simulink library "DSCA"  (R2016b)
settings: Solver=VariableStepAuto  StartTime=0.0  StopTime=10.0  RelTol=1e-3
undefined symbols (not defined in the file): CAL_FilterResetThd, CAL_MeasNoiseVelKF, CAL_mm_PER_tick, CAL_NORTH, CAL_procNoiseVelKF, CAL_ROBO_LENG, CAL_WheelDiameter_cm, CONST_EnableDelay, CONST_EndOfLineEnableFlg, ENU_BACKWARD, ENU_DIAG, ENU_FORWARD, ENU_STOP, gearRatio
libraries: movingAverage_1ms_to_5ms x5, simulink_need_slupdate x2, MotorModelDiscreteTf x2, ThetaOverFlowFilter x1
settings Model: Creator=oelkawok  LastModifiedBy=oelkawok

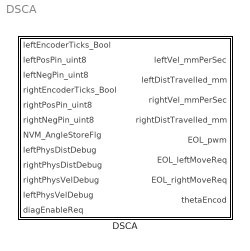
== system DSCA ==
  DSCA : Subsystem  TreatAsAtomicUnit=on

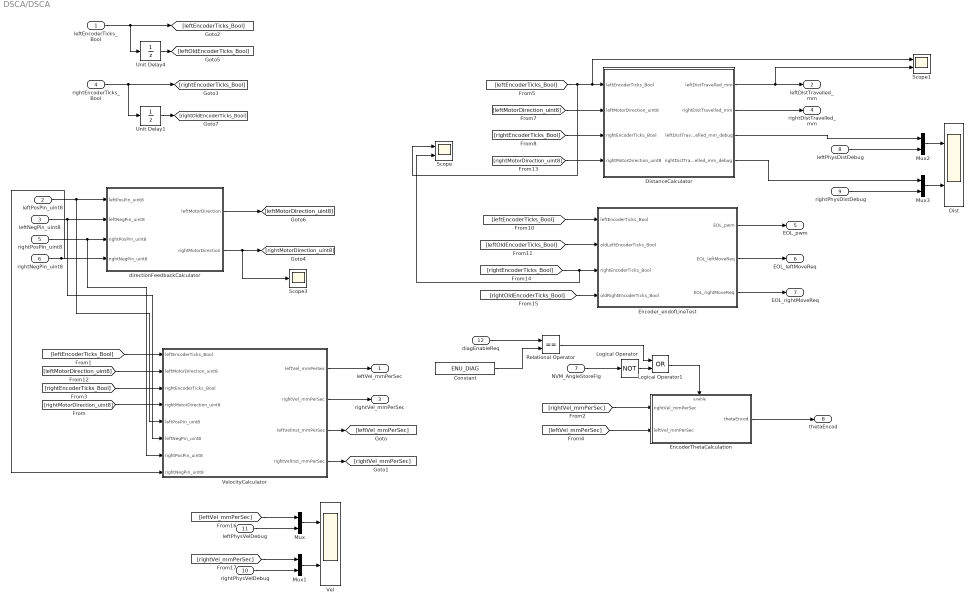
== system DSCA/DSCA ==
  leftEncoderTicks_Bool : Inport
  leftPosPin_uint8 : Inport  Port=2
  leftNegPin_uint8 : Inport  Port=3
  rightEncoderTicks_Bool : Inport  Port=4
  rightPosPin_uint8 : Inport  Port=5
  rightNegPin_uint8 : Inport  Port=6
  NVM_AngleStoreFlg : Inport  Port=7
  leftPhysDistDebug : Inport  Port=8
  rightPhysDistDebug : Inport  Port=9
  rightPhysVelDebug : Inport  Port=10
  leftPhysVelDebug : Inport  Port=11
  diagEnableReq : Inport  Port=12
  Constant : Constant  Value=ENU_DIAG
  Dist : Scope  NumInputPorts=2
  DistanceCalculator : Subsystem
  EncoderThetaCalculation : Subsystem
  Encoder_endofLineTest : Subsystem
  Logical Operator : Logic  Operator=NOT  IconShape=distinctive  AllPortsSameDT=off  OutDataTypeStr=boolean
  Logical Operator1 : Logic  Operator=OR  AllPortsSameDT=off  OutDataTypeStr=boolean
  Mux{,1..3} (4 alike) : Mux  Inputs=2
  Relational Operator : RelationalOperator  Operator===  OutDataTypeStr=boolean  RndMeth=Simplest
  Scope : Scope  NumInputPorts=2
  Scope1 : Scope  NumInputPorts=2
  Scope3 : Scope
  Unit Delay1 : UnitDelay  SampleTime=-1
      settings: AttributesFormatString=Init: %<InitialCondition>
  Unit Delay4 : UnitDelay  SampleTime=-1
      settings: AttributesFormatString=Init: %<InitialCondition>
  Vel : Scope  NumInputPorts=2
  VelocityCalculator : Subsystem
  directionFeedbackCalculator : Subsystem
  leftVel_mmPerSec : Outport
  leftDistTravelled_mm : Outport  Port=2
  rightVel_mmPerSec : Outport  Port=3
  rightDistTravelled_mm : Outport  Port=4
  EOL_pwm : Outport  Port=5
  EOL_leftMoveReq : Outport  Port=6
  EOL_rightMoveReq : Outport  Port=7
  thetaEncod : Outport  Port=8
  wires:
  Relational Operator/1 -> Logical Operator1/1
  Constant/1 -> Relational Operator/2
  diagEnableReq/1 -> Relational Operator/1
  Logical Operator1/1 -> EncoderThetaCalculation/Enable
  Logical Operator/1 -> Logical Operator1/2
  VelocityCalculator/2(rightVel_mmPerSec) -> rightVel_mmPerSec/1
  VelocityCalculator/1(leftVel_mmPerSec) -> leftVel_mmPerSec/1
  EncoderThetaCalculation/1(thetaEncod) -> thetaEncod/1
  rightPhysVelDebug/1 -> Mux1/2
  leftPhysVelDebug/1 -> Mux/2
  [rightVel_mmPerSec] -> Mux1/1
  [leftVel_mmPerSec] -> Mux/1
  [rightVel_mmPerSec] -> EncoderThetaCalculation/1(rightVel_mmPerSec)
  [leftVel_mmPerSec] -> EncoderThetaCalculation/2(leftVel_mmPerSec)
  VelocityCalculator/3(leftVelInst_mmPerSec) -> [leftVel_mmPerSec]
  VelocityCalculator/4(rightVelInst_mmPerSec) -> [rightVel_mmPerSec]
  rightPhysDistDebug/1 -> Mux3/2
  DistanceCalculator/4(rightDistTravelled_mm_debug) -> Mux3/1
  Mux3/1 -> Dist/2
  Mux2/1 -> Dist/1
  [rightMotorDirection_uint8] -> VelocityCalculator/4(rightMotorDirection_uint8)
  Mux1/1 -> Vel/2
  Mux/1 -> Vel/1
  leftPhysDistDebug/1 -> Mux2/2
  DistanceCalculator/3(leftDistTravelled_mm_debug) -> Mux2/1
  NVM_AngleStoreFlg/1 -> Logical Operator/1
  Encoder_endofLineTest/1(EOL_pwm) -> EOL_pwm/1
  Encoder_endofLineTest/2(EOL_leftMoveReq) -> EOL_leftMoveReq/1
  Encoder_endofLineTest/3(EOL_rightMoveReq) -> EOL_rightMoveReq/1
  [rightOldEncoderTicks_Bool] -> Encoder_endofLineTest/4(oldRightEncoderTicks_Bool)
  [rightEncoderTicks_Bool] -> Encoder_endofLineTest/3(rightEncoderTicks_Bool), Scope/2
  [leftOldEncoderTicks_Bool] -> Encoder_endofLineTest/2(oldLeftEncoderTicks_Bool)
  [leftEncoderTicks_Bool] -> Encoder_endofLineTest/1(leftEncoderTicks_Bool)
  [rightEncoderTicks_Bool] -> DistanceCalculator/3(rightEncoderTicks_Bool)
  [leftEncoderTicks_Bool] -> DistanceCalculator/1(leftEncoderTicks_Bool), Scope1/1, Scope/1
  [rightEncoderTicks_Bool] -> VelocityCalculator/3(rightEncoderTicks_Bool)
  [leftEncoderTicks_Bool] -> VelocityCalculator/1(leftEncoderTicks_Bool)
  Unit Delay4/1 -> [leftOldEncoderTicks_Bool]
  Unit Delay1/1 -> [rightOldEncoderTicks_Bool]
  leftEncoderTicks_Bool/1 -> Unit Delay4/1, [leftEncoderTicks_Bool]
  rightEncoderTicks_Bool/1 -> [rightEncoderTicks_Bool], Unit Delay1/1
  [leftMotorDirection_uint8] -> VelocityCalculator/2(leftMotorDirection_uint8)
  DistanceCalculator/2(rightDistTravelled_mm) -> rightDistTravelled_mm/1
  [rightMotorDirection_uint8] -> DistanceCalculator/4(rightMotorDirection_uint8)
  [leftMotorDirection_uint8] -> DistanceCalculator/2(leftMotorDirection_uint8)
  DistanceCalculator/1(leftDistTravelled_mm) -> leftDistTravelled_mm/1, Scope1/2
  directionFeedbackCalculator/2(rightMotorDirection) -> [rightMotorDirection_uint8], Scope3/1
  rightNegPin_uint8/1 -> directionFeedbackCalculator/4(rightNegPin_uint8), VelocityCalculator/8(rightNegPin_uint8)
  rightPosPin_uint8/1 -> directionFeedbackCalculator/3(rightPosPin_uint8), VelocityCalculator/7(rightPosPin_uint8)
  directionFeedbackCalculator/1(leftMotorDirection) -> [leftMotorDirection_uint8]
  leftNegPin_uint8/1 -> directionFeedbackCalculator/2(leftNegPin_uint8), VelocityCalculator/6(leftNegPin_uint8)
  leftPosPin_uint8/1 -> directionFeedbackCalculator/1(leftPosPin_uint8), VelocityCalculator/5(leftPosPin_uint8)

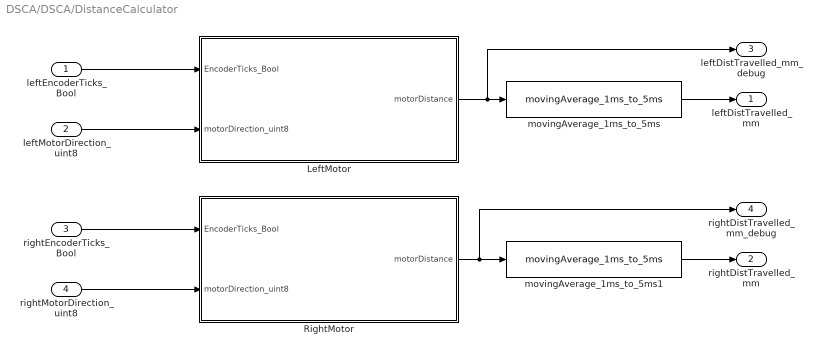
== system DSCA/DSCA/DistanceCalculator ==
  leftEncoderTicks_Bool : Inport
  leftMotorDirection_uint8 : Inport  Port=2
  rightEncoderTicks_Bool : Inport  Port=3
  rightMotorDirection_uint8 : Inport  Port=4
  LeftMotor : Subsystem
  RightMotor : Subsystem
  movingAverage_1ms_to_5ms : movingAverage_1ms_to_5ms/movingAverage_1ms_to_5ms
  movingAverage_1ms_to_5ms1 : movingAverage_1ms_to_5ms/movingAverage_1ms_to_5ms
  leftDistTravelled_mm : Outport
  rightDistTravelled_mm : Outport  Port=2
  leftDistTravelled_mm_debug : Outport  Port=3
  rightDistTravelled_mm_debug : Outport  Port=4
  wires:
  rightMotorDirection_uint8/1 -> RightMotor/2(motorDirection_uint8)
  rightEncoderTicks_Bool/1 -> RightMotor/1(EncoderTicks_Bool)
  leftMotorDirection_uint8/1 -> LeftMotor/2(motorDirection_uint8)
  leftEncoderTicks_Bool/1 -> LeftMotor/1(EncoderTicks_Bool)
  movingAverage_1ms_to_5ms/1 -> leftDistTravelled_mm/1
  LeftMotor/1(motorDistance) -> leftDistTravelled_mm_debug/1, movingAverage_1ms_to_5ms/1
  movingAverage_1ms_to_5ms1/1 -> rightDistTravelled_mm/1
  RightMotor/1(motorDistance) -> rightDistTravelled_mm_debug/1, movingAverage_1ms_to_5ms1/1

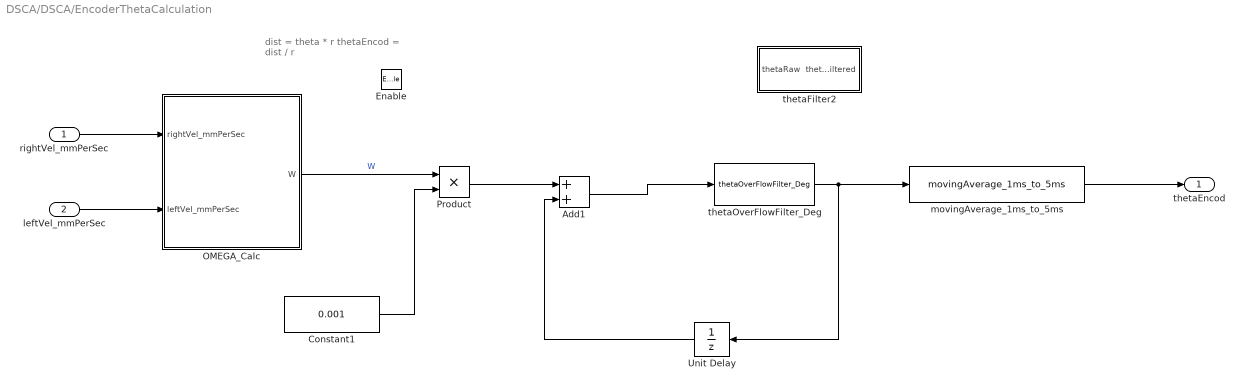
== system DSCA/DSCA/EncoderThetaCalculation ==
  note: dist = theta * r
      | thetaEncod = dist / r
  rightVel_mmPerSec : Inport
  leftVel_mmPerSec : Inport  Port=2
  Enable : EnablePort
  Add1 : Sum
  Constant1 : Constant  Value=0.001
  OMEGA_Calc : Subsystem
  Product : Product
  Unit Delay : UnitDelay  InitialCondition=CAL_NORTH  SampleTime=-1
  movingAverage_1ms_to_5ms : movingAverage_1ms_to_5ms/movingAverage_1ms_to_5ms
  thetaFilter2 : Subsystem
  thetaOverFlowFilter_Deg : ThetaOverFlowFilter/thetaOverFlowFilter_Deg
  thetaEncod : Outport
  wires:
  movingAverage_1ms_to_5ms/1 -> thetaEncod/1
  Unit Delay/1 -> Add1/2
  Add1/1 -> thetaOverFlowFilter_Deg/1
  Product/1 -> Add1/1
  thetaOverFlowFilter_Deg/1 -> Unit Delay/1, movingAverage_1ms_to_5ms/1
  rightVel_mmPerSec/1 -> OMEGA_Calc/1(rightVel_mmPerSec)
  leftVel_mmPerSec/1 -> OMEGA_Calc/2(leftVel_mmPerSec)
  OMEGA_Calc/1(W) -> Product/1  "W"
  Constant1/1 -> Product/2

== system DSCA/DSCA/Encoder_endofLineTest ==
  leftEncoderTicks_Bool : Inport
  oldLeftEncoderTicks_Bool : Inport  Port=2
  rightEncoderTicks_Bool : Inport  Port=3
  oldRightEncoderTicks_Bool : Inport  Port=4
  CONST_EndOfLineEnableFlg : Constant  Value=CONST_EndOfLineEnableFlg
  endofLineTest : Subsystem
  EOL_pwm : Outport
  EOL_leftMoveReq : Outport  Port=2
  EOL_rightMoveReq : Outport  Port=3
  wires:
  endofLineTest/2(EOL_leftMoveReq) -> EOL_leftMoveReq/1
  endofLineTest/3(EOL_rightMoveReq) -> EOL_rightMoveReq/1
  oldRightEncoderTicks_Bool/1 -> endofLineTest/4(oldRightEncoderTicks_Bool)
  rightEncoderTicks_Bool/1 -> endofLineTest/3(rightEncoderTicks_Bool)
  leftEncoderTicks_Bool/1 -> endofLineTest/1(leftEncoderTicks_Bool)
  oldLeftEncoderTicks_Bool/1 -> endofLineTest/2(oldLeftEncoderTicks_Bool)
  endofLineTest/1(EOL_pwm) -> EOL_pwm/1
  CONST_EndOfLineEnableFlg/1 -> endofLineTest/Enable

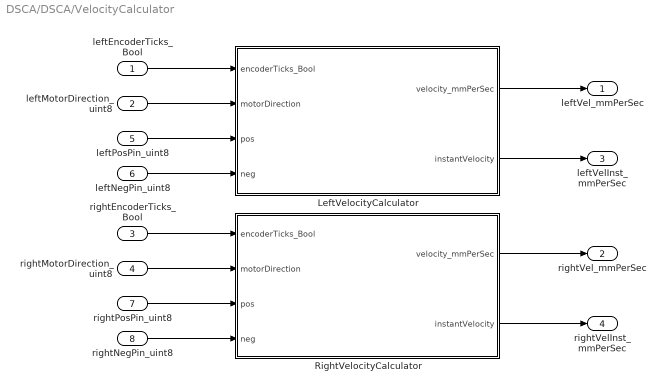
== system DSCA/DSCA/VelocityCalculator ==
  leftEncoderTicks_Bool : Inport
  leftMotorDirection_uint8 : Inport  Port=2
  rightEncoderTicks_Bool : Inport  Port=3
  rightMotorDirection_uint8 : Inport  Port=4
  leftPosPin_uint8 : Inport  Port=5
  leftNegPin_uint8 : Inport  Port=6
  rightPosPin_uint8 : Inport  Port=7
  rightNegPin_uint8 : Inport  Port=8
  LeftVelocityCalculator : Subsystem
  RightVelocityCalculator : Subsystem
  leftVel_mmPerSec : Outport
  rightVel_mmPerSec : Outport  Port=2
  leftVelInst_mmPerSec : Outport  Port=3
  rightVelInst_mmPerSec : Outport  Port=4
  wires:
  rightNegPin_uint8/1 -> RightVelocityCalculator/4(neg)
  rightPosPin_uint8/1 -> RightVelocityCalculator/3(pos)
  leftNegPin_uint8/1 -> LeftVelocityCalculator/4(neg)
  leftPosPin_uint8/1 -> LeftVelocityCalculator/3(pos)
  RightVelocityCalculator/2(instantVelocity) -> rightVelInst_mmPerSec/1
  LeftVelocityCalculator/2(instantVelocity) -> leftVelInst_mmPerSec/1
  leftMotorDirection_uint8/1 -> LeftVelocityCalculator/2(motorDirection)
  rightMotorDirection_uint8/1 -> RightVelocityCalculator/2(motorDirection)
  LeftVelocityCalculator/1(velocity_mmPerSec) -> leftVel_mmPerSec/1
  leftEncoderTicks_Bool/1 -> LeftVelocityCalculator/1(encoderTicks_Bool)
  RightVelocityCalculator/1(velocity_mmPerSec) -> rightVel_mmPerSec/1
  rightEncoderTicks_Bool/1 -> RightVelocityCalculator/1(encoderTicks_Bool)

== system DSCA/DSCA/directionFeedbackCalculator ==
  leftPosPin_uint8 : Inport
  leftNegPin_uint8 : Inport  Port=2
  rightPosPin_uint8 : Inport  Port=3
  rightNegPin_uint8 : Inport  Port=4
  LeftMotor : Subsystem
  RightMotor : Subsystem
  leftMotorDirection : Outport
  rightMotorDirection : Outport  Port=2
  wires:
  RightMotor/1(MotorDirection) -> rightMotorDirection/1
  rightNegPin_uint8/1 -> RightMotor/2(NegPin_uint8)
  rightPosPin_uint8/1 -> RightMotor/1(PosPin_uint8)
  LeftMotor/1(MotorDirection) -> leftMotorDirection/1
  leftNegPin_uint8/1 -> LeftMotor/2(NegPin_uint8)
  leftPosPin_uint8/1 -> LeftMotor/1(PosPin_uint8)

== system DSCA/DSCA/DistanceCalculator/LeftMotor ==
  EncoderTicks_Bool : Inport
  motorDirection_uint8 : Inport  Port=2
  Data Type Conversion : DataTypeConversion  OutDataTypeStr=single
  EncoderIncrement : Subsystem  TreatAsAtomicUnit=on
  Gain1 : Gain  Gain=CAL_mm_PER_tick
  motorDistance : Outport
  wires:
  motorDirection_uint8/1 -> EncoderIncrement/1(motorDirection)
  EncoderTicks_Bool/1 -> EncoderIncrement/Trigger
  EncoderIncrement/1(distCounter) -> Data Type Conversion/1
  Gain1/1 -> motorDistance/1
  Data Type Conversion/1 -> Gain1/1

== system DSCA/DSCA/DistanceCalculator/RightMotor ==
  EncoderTicks_Bool : Inport
  motorDirection_uint8 : Inport  Port=2
  Data Type Conversion : DataTypeConversion  OutDataTypeStr=single
  EncoderIncrement : Subsystem  TreatAsAtomicUnit=on
  Gain1 : Gain  Gain=CAL_mm_PER_tick
  motorDistance : Outport
  wires:
  Data Type Conversion/1 -> Gain1/1
  Gain1/1 -> motorDistance/1
  EncoderIncrement/1(distCounter) -> Data Type Conversion/1
  EncoderTicks_Bool/1 -> EncoderIncrement/Trigger
  motorDirection_uint8/1 -> EncoderIncrement/1(motorDirection)

== system DSCA/DSCA/EncoderThetaCalculation/OMEGA_Calc ==
  rightVel_mmPerSec : Inport
  leftVel_mmPerSec : Inport  Port=2
  Add : Sum  Inputs=+-
  Constant3 : Constant  Value=CAL_ROBO_LENG
  Divide1 : Product  Inputs=*/  OutDataTypeStr=single
  W : Outport
  wires:
  rightVel_mmPerSec/1 -> Add/2
  leftVel_mmPerSec/1 -> Add/1
  Add/1 -> Divide1/1
  Divide1/1 -> W/1
  Constant3/1 -> Divide1/2

== system DSCA/DSCA/EncoderThetaCalculation/thetaFilter2 ==
  thetaRaw : Inport
  Add : Sum  Inputs=+-
  Add1 : Sum
  Constant : Constant  Value=360
  Constant1 : Constant  Value=360
  Constant2 : Constant  Value=0
  Relational Operator : RelationalOperator  Operator=>  OutDataTypeStr=boolean  RndMeth=Nearest
  Relational Operator1 : RelationalOperator  Operator=<  OutDataTypeStr=boolean  RndMeth=Nearest
  Switch : Switch  Criteria=u2 > Threshold
  Switch1 : Switch  Criteria=u2 > Threshold
  thetaFiltered : Outport
  wires:
  thetaRaw/1 -> Switch1/3, Add/1, Add1/2, Relational Operator1/1, Relational Operator/1
  Constant/1 -> Add1/1, Relational Operator/2
  Relational Operator/1 -> Switch/2
  Constant1/1 -> Add/2
  Add/1 -> Switch/1
  Constant2/1 -> Relational Operator1/2
  Relational Operator1/1 -> Switch1/2
  Add1/1 -> Switch1/1
  Switch1/1 -> Switch/3
  Switch/1 -> thetaFiltered/1

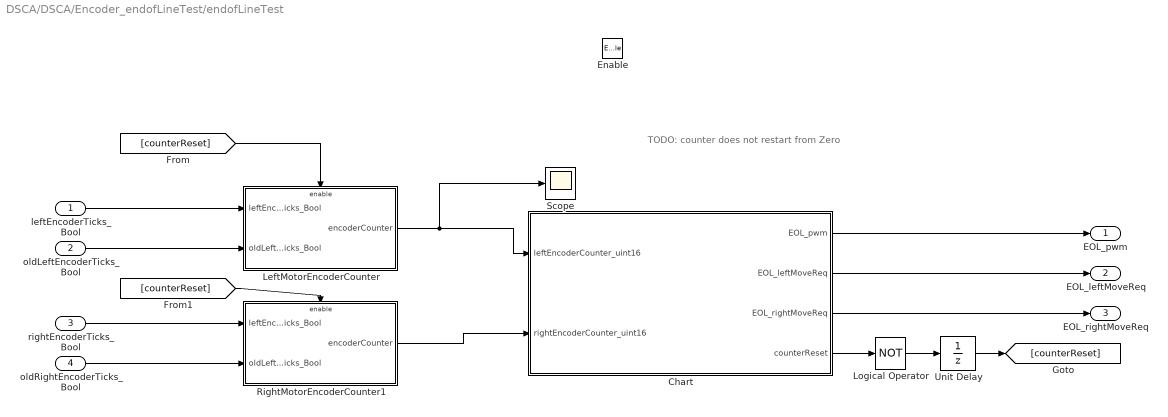
== system DSCA/DSCA/Encoder_endofLineTest/endofLineTest ==
  note: TODO: counter does not restart from Zero
  leftEncoderTicks_Bool : Inport
  oldLeftEncoderTicks_Bool : Inport  Port=2
  rightEncoderTicks_Bool : Inport  Port=3
  oldRightEncoderTicks_Bool : Inport  Port=4
  Enable : EnablePort
  Chart : Stateflow chart  TreatAsAtomicUnit=on
  LeftMotorEncoderCounter : Subsystem
  Logical Operator : Logic  Operator=NOT  Inputs=NOT  IconShape=distinctive  AllPortsSameDT=off  OutDataTypeStr=boolean
  RightMotorEncoderCounter1 : Subsystem
  Scope : Scope
  Unit Delay : UnitDelay  InitialCondition=1  SampleTime=-1
  EOL_pwm : Outport
  EOL_leftMoveReq : Outport  Port=2
  EOL_rightMoveReq : Outport  Port=3
  wires:
  LeftMotorEncoderCounter/1(encoderCounter) -> Chart/1(leftEncoderCounter_uint16), Scope/1
  Unit Delay/1 -> [counterReset]
  Chart/3(EOL_rightMoveReq) -> EOL_rightMoveReq/1
  Chart/2(EOL_leftMoveReq) -> EOL_leftMoveReq/1
  Chart/1(EOL_pwm) -> EOL_pwm/1
  Logical Operator/1 -> Unit Delay/1
  [counterReset] -> LeftMotorEncoderCounter/Enable
  [counterReset] -> RightMotorEncoderCounter1/Enable
  Chart/4(counterReset) -> Logical Operator/1
  RightMotorEncoderCounter1/1(encoderCounter) -> Chart/2(rightEncoderCounter_uint16)
  rightEncoderTicks_Bool/1 -> RightMotorEncoderCounter1/1(leftEncoderTicks_Bool)
  oldRightEncoderTicks_Bool/1 -> RightMotorEncoderCounter1/2(oldLeftEncoderTicks_Bool)
  oldLeftEncoderTicks_Bool/1 -> LeftMotorEncoderCounter/2(oldLeftEncoderTicks_Bool)
  leftEncoderTicks_Bool/1 -> LeftMotorEncoderCounter/1(leftEncoderTicks_Bool)

== system DSCA/DSCA/VelocityCalculator/LeftVelocityCalculator ==
  encoderTicks_Bool : Inport
  motorDirection : Inport  Port=2
  pos : Inport  Port=3
  neg : Inport  Port=4
  LeftMotor : Subsystem
  movingAverage_1ms_to_5ms : movingAverage_1ms_to_5ms/movingAverage_1ms_to_5ms
  velocity_mmPerSec : Outport
  instantVelocity : Outport  Port=2
  wires:
  neg/1 -> LeftMotor/4(neg)
  pos/1 -> LeftMotor/3(pos)
  movingAverage_1ms_to_5ms/1 -> velocity_mmPerSec/1
  LeftMotor/1(motorSpd) -> instantVelocity/1, movingAverage_1ms_to_5ms/1
  motorDirection/1 -> LeftMotor/2(motorDirection_uint8)
  encoderTicks_Bool/1 -> LeftMotor/1(EncoderTicks_Bool)

== system DSCA/DSCA/VelocityCalculator/RightVelocityCalculator ==
  encoderTicks_Bool : Inport
  motorDirection : Inport  Port=2
  pos : Inport  Port=3
  neg : Inport  Port=4
  LeftMotor : Subsystem
  movingAverage_1ms_to_5ms : movingAverage_1ms_to_5ms/movingAverage_1ms_to_5ms
  velocity_mmPerSec : Outport
  instantVelocity : Outport  Port=2
  wires:
  neg/1 -> LeftMotor/4(neg)
  pos/1 -> LeftMotor/3(pos)
  movingAverage_1ms_to_5ms/1 -> velocity_mmPerSec/1
  encoderTicks_Bool/1 -> LeftMotor/1(EncoderTicks_Bool)
  LeftMotor/1(motorSpd) -> instantVelocity/1, movingAverage_1ms_to_5ms/1
  motorDirection/1 -> LeftMotor/2(motorDirection_uint8)

== system DSCA/DSCA/directionFeedbackCalculator/LeftMotor ==
  PosPin_uint8 : Inport
  NegPin_uint8 : Inport  Port=2
  Constant13 : Constant  Value=ENU_STOP
  Constant14 : Constant  Value=ENU_BACKWARD
  Constant15 : Constant  Value=ENU_FORWARD
  Relational Operator5 : RelationalOperator  Operator=>  OutDataTypeStr=boolean  RndMeth=Simplest
  Relational Operator6 : RelationalOperator  Operator=<  OutDataTypeStr=boolean  RndMeth=Simplest
  Switch5 : Switch  Criteria=u2 ~= 0
  Switch6 : Switch  Criteria=u2 ~= 0
  MotorDirection : Outport
  wires:
  NegPin_uint8/1 -> Relational Operator5/2, Relational Operator6/2
  Relational Operator5/1 -> Switch5/2
  PosPin_uint8/1 -> Relational Operator5/1, Relational Operator6/1
  Constant14/1 -> Switch6/1
  Constant13/1 -> Switch6/3
  Constant15/1 -> Switch5/1
  Relational Operator6/1 -> Switch6/2
  Switch6/1 -> Switch5/3
  Switch5/1 -> MotorDirection/1

== system DSCA/DSCA/directionFeedbackCalculator/RightMotor ==
  PosPin_uint8 : Inport
  NegPin_uint8 : Inport  Port=2
  Constant13 : Constant  Value=ENU_STOP
  Constant14 : Constant  Value=ENU_BACKWARD
  Constant15 : Constant  Value=ENU_FORWARD
  Relational Operator5 : RelationalOperator  Operator=>  OutDataTypeStr=boolean  RndMeth=Simplest
  Relational Operator6 : RelationalOperator  Operator=<  OutDataTypeStr=boolean  RndMeth=Simplest
  Switch5 : Switch  Criteria=u2 ~= 0
  Switch6 : Switch  Criteria=u2 ~= 0
  MotorDirection : Outport
  wires:
  Switch5/1 -> MotorDirection/1
  Switch6/1 -> Switch5/3
  Relational Operator6/1 -> Switch6/2
  Constant15/1 -> Switch5/1
  Constant13/1 -> Switch6/3
  Constant14/1 -> Switch6/1
  PosPin_uint8/1 -> Relational Operator6/1, Relational Operator5/1
  Relational Operator5/1 -> Switch5/2
  NegPin_uint8/1 -> Relational Operator6/2, Relational Operator5/2

== system DSCA/DSCA/DistanceCalculator/LeftMotor/EncoderIncrement ==
  motorDirection : Inport
  function : TriggerPort  VariantControl=Variant
  Add : Sum
  Constant1 : Constant  Value=int32(1)
  Constant2 : Constant  Value=int32(-1)
  Constant6 : Constant  Value=ENU_FORWARD
  Relational Operator : RelationalOperator  Operator===  OutDataTypeStr=boolean  RndMeth=Simplest
  Switch1 : Switch  Criteria=u2 ~= 0
  Unit Delay : UnitDelay  SampleTime=-1
  distCounter : Outport
  wires:
  Constant1/1 -> Switch1/1
  Constant6/1 -> Relational Operator/2
  Relational Operator/1 -> Switch1/2
  motorDirection/1 -> Relational Operator/1
  Constant2/1 -> Switch1/3
  Switch1/1 -> Add/2
  Add/1 -> distCounter/1, Unit Delay/1
  Unit Delay/1 -> Add/1

== system DSCA/DSCA/DistanceCalculator/RightMotor/EncoderIncrement ==
  motorDirection : Inport
  function : TriggerPort  VariantControl=Variant
  Add : Sum
  Constant1 : Constant  Value=int32(1)
  Constant2 : Constant  Value=int32(-1)
  Constant6 : Constant  Value=ENU_FORWARD
  Relational Operator : RelationalOperator  Operator===  OutDataTypeStr=boolean  RndMeth=Simplest
  Switch1 : Switch  Criteria=u2 ~= 0
  Unit Delay : UnitDelay  SampleTime=-1
  distCounter : Outport
  wires:
  Unit Delay/1 -> Add/1
  Add/1 -> Unit Delay/1, distCounter/1
  Switch1/1 -> Add/2
  Constant2/1 -> Switch1/3
  motorDirection/1 -> Relational Operator/1
  Relational Operator/1 -> Switch1/2
  Constant6/1 -> Relational Operator/2
  Constant1/1 -> Switch1/1

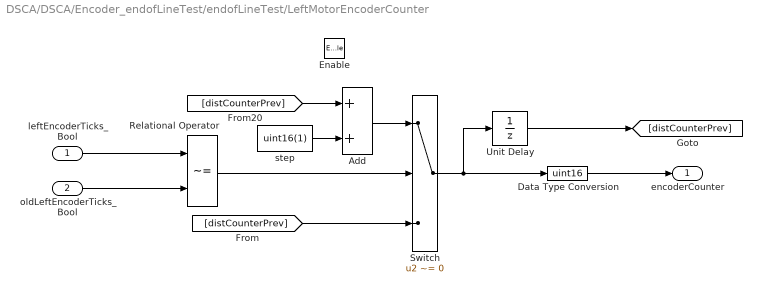
== system DSCA/DSCA/Encoder_endofLineTest/endofLineTest/LeftMotorEncoderCounter ==
  leftEncoderTicks_Bool : Inport
  oldLeftEncoderTicks_Bool : Inport  Port=2
  Enable : EnablePort  StatesWhenEnabling=reset
  Add : Sum
  Data Type Conversion : DataTypeConversion  OutDataTypeStr=uint16
  Relational Operator : RelationalOperator  Operator=~=  OutDataTypeStr=boolean  RndMeth=Simplest
  Switch : Switch  Criteria=u2 ~= 0
  Unit Delay : UnitDelay  SampleTime=-1
  step : Constant  Value=uint16(1)  OutDataTypeStr=single
  encoderCounter : Outport  OutputWhenDisabled=reset  InitialOutput=0
  wires:
  Data Type Conversion/1 -> encoderCounter/1
  oldLeftEncoderTicks_Bool/1 -> Relational Operator/2
  leftEncoderTicks_Bool/1 -> Relational Operator/1
  Switch/1 -> Unit Delay/1, Data Type Conversion/1
  [distCounterPrev] -> Switch/3
  step/1 -> Add/2
  [distCounterPrev] -> Add/1
  Relational Operator/1 -> Switch/2
  Add/1 -> Switch/1
  Unit Delay/1 -> [distCounterPrev]

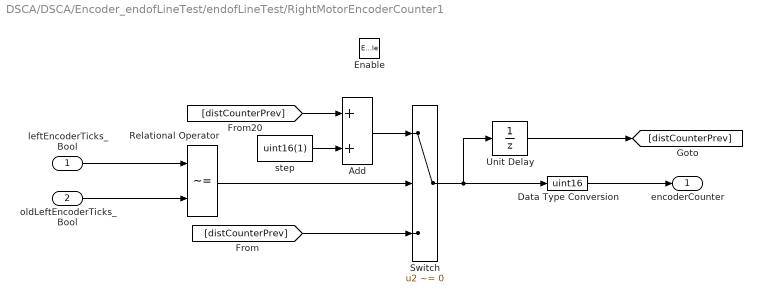
== system DSCA/DSCA/Encoder_endofLineTest/endofLineTest/RightMotorEncoderCounter1 ==
  leftEncoderTicks_Bool : Inport
  oldLeftEncoderTicks_Bool : Inport  Port=2
  Enable : EnablePort  StatesWhenEnabling=reset
  Add : Sum
  Data Type Conversion : DataTypeConversion  OutDataTypeStr=uint16
  Relational Operator : RelationalOperator  Operator=~=  OutDataTypeStr=boolean  RndMeth=Simplest
  Switch : Switch  Criteria=u2 ~= 0
  Unit Delay : UnitDelay  SampleTime=-1
  step : Constant  Value=uint16(1)  OutDataTypeStr=single
  encoderCounter : Outport  OutputWhenDisabled=reset  InitialOutput=0
  wires:
  Unit Delay/1 -> [distCounterPrev]
  Add/1 -> Switch/1
  Relational Operator/1 -> Switch/2
  [distCounterPrev] -> Add/1
  step/1 -> Add/2
  [distCounterPrev] -> Switch/3
  Switch/1 -> Data Type Conversion/1, Unit Delay/1
  leftEncoderTicks_Bool/1 -> Relational Operator/1
  oldLeftEncoderTicks_Bool/1 -> Relational Operator/2
  Data Type Conversion/1 -> encoderCounter/1

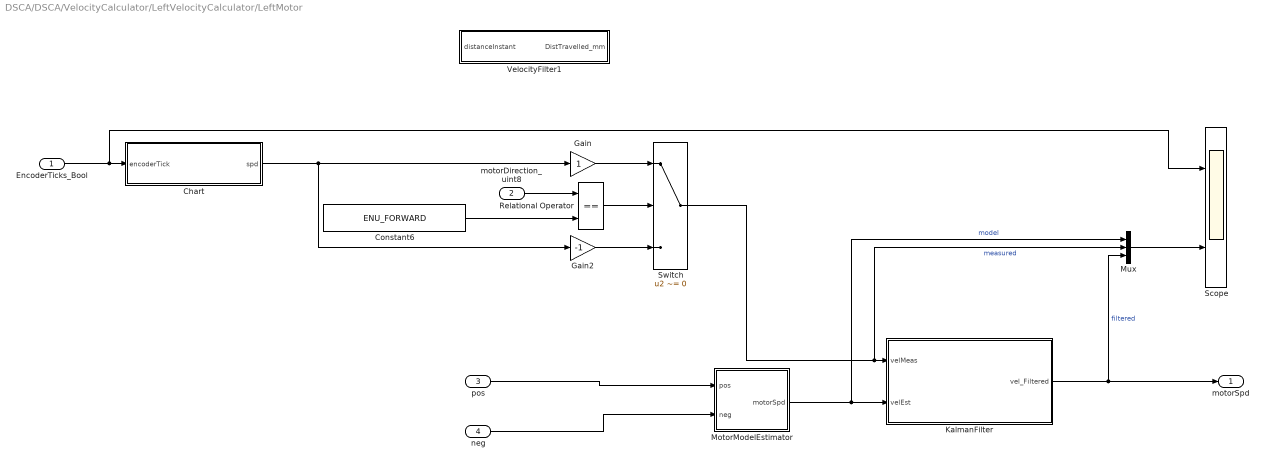
== system DSCA/DSCA/VelocityCalculator/LeftVelocityCalculator/LeftMotor ==
  EncoderTicks_Bool : Inport
  motorDirection_uint8 : Inport  Port=2
  pos : Inport  Port=3
  neg : Inport  Port=4
  Chart : Stateflow chart  TreatAsAtomicUnit=on
  Constant6 : Constant  Value=ENU_FORWARD
  Gain : Gain
  Gain2 : Gain  Gain=-1
  KalmanFilter : Subsystem
  MotorModelEstimator : Subsystem
  Mux : Mux  Inputs=3
  Relational Operator : RelationalOperator  Operator===  OutDataTypeStr=boolean  RndMeth=Simplest
  Scope : Scope  NumInputPorts=2
  Switch : Switch  Criteria=u2 ~= 0
  VelocityFilter1 : Subsystem
  motorSpd : Outport
  wires:
  Mux/1 -> Scope/2
  KalmanFilter/1(" vel_Filtered") -> motorSpd/1, Mux/3  "filtered"
  neg/1 -> MotorModelEstimator/2(neg)
  pos/1 -> MotorModelEstimator/1(pos)
  MotorModelEstimator/1(motorSpd) -> KalmanFilter/2(velEst), Mux/1  "model"
  Chart/1(spd) -> Gain/1, Gain2/1
  Switch/1 -> KalmanFilter/1(velMeas), Mux/2  "measured"
  Constant6/1 -> Relational Operator/2
  Gain2/1 -> Switch/3
  Gain/1 -> Switch/1
  Relational Operator/1 -> Switch/2
  motorDirection_uint8/1 -> Relational Operator/1
  EncoderTicks_Bool/1 -> Chart/1(encoderTick), Scope/1

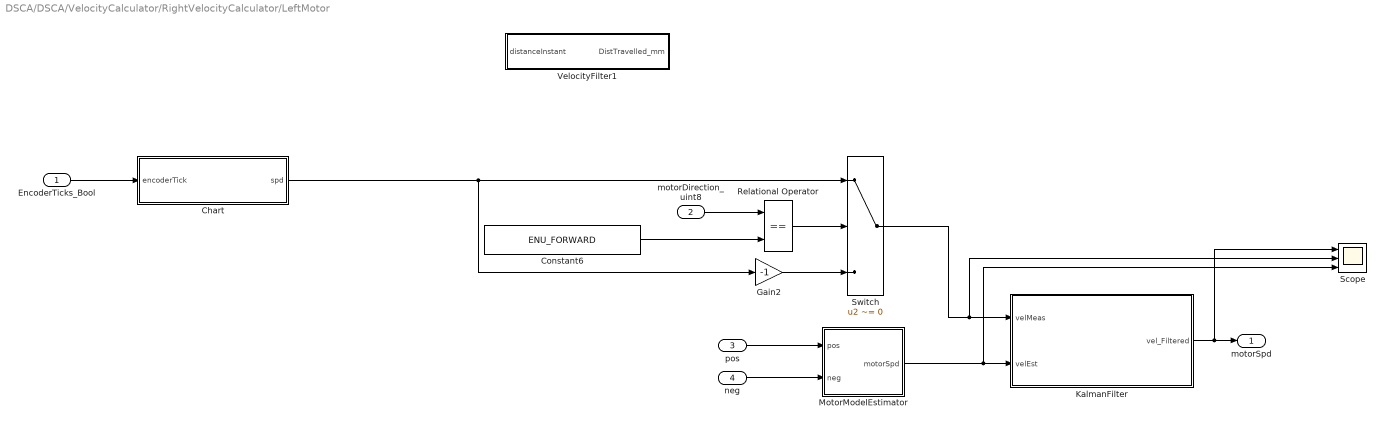
== system DSCA/DSCA/VelocityCalculator/RightVelocityCalculator/LeftMotor ==
  EncoderTicks_Bool : Inport
  motorDirection_uint8 : Inport  Port=2
  pos : Inport  Port=3
  neg : Inport  Port=4
  Chart : Stateflow chart  TreatAsAtomicUnit=on
  Constant6 : Constant  Value=ENU_FORWARD
  Gain2 : Gain  Gain=-1
  KalmanFilter : Subsystem
  MotorModelEstimator : Subsystem
  Relational Operator : RelationalOperator  Operator===  OutDataTypeStr=boolean  RndMeth=Simplest
  Scope : Scope  NumInputPorts=3
  Switch : Switch  Criteria=u2 ~= 0
  VelocityFilter1 : Subsystem
  motorSpd : Outport
  wires:
  KalmanFilter/1(" vel_Filtered") -> motorSpd/1, Scope/1
  Switch/1 -> KalmanFilter/1(velMeas), Scope/2
  MotorModelEstimator/1(motorSpd) -> KalmanFilter/2(velEst), Scope/3
  neg/1 -> MotorModelEstimator/2(neg)
  pos/1 -> MotorModelEstimator/1(pos)
  EncoderTicks_Bool/1 -> Chart/1(encoderTick)
  motorDirection_uint8/1 -> Relational Operator/1
  Relational Operator/1 -> Switch/2
  Chart/1(spd) -> Gain2/1, Switch/1
  Gain2/1 -> Switch/3
  Constant6/1 -> Relational Operator/2

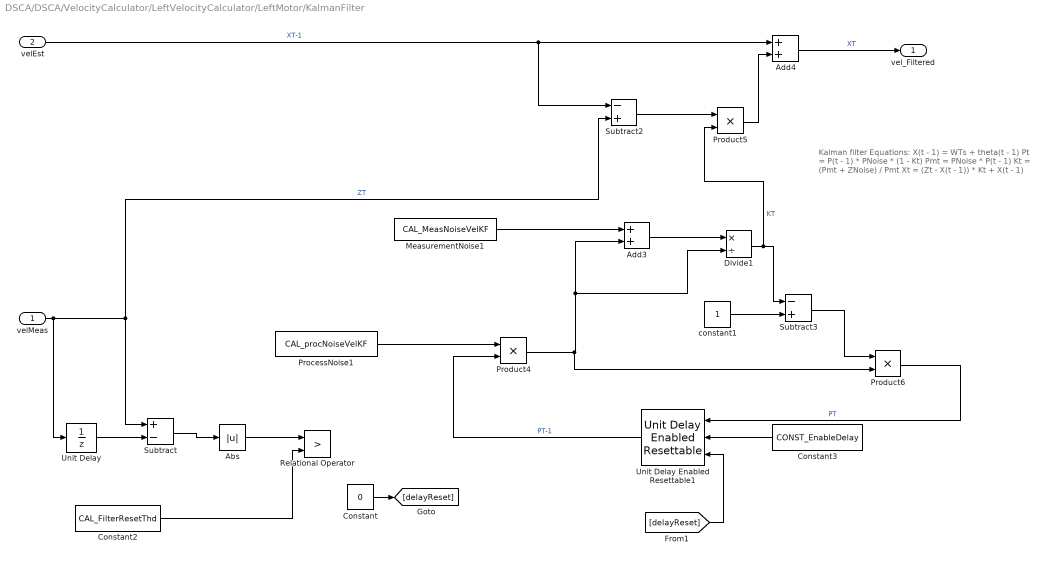
== system DSCA/DSCA/VelocityCalculator/LeftVelocityCalculator/LeftMotor/KalmanFilter ==
  note: Kalman filter Equations:
      | X(t - 1) = WTs + theta(t - 1)
      | Pt = P(t - 1) * PNoise * (1 - Kt)
      | Pmt = PNoise * P(t - 1)
      | Kt = (Pmt + ZNoise) / Pmt
      | Xt = (Zt - X(t - 1)) * Kt + X(t - 1)
  velMeas : Inport
  velEst : Inport  Port=2
  Abs : Abs
  Add3 : Sum
  Add4 : Sum  OutDataTypeStr=single
  Constant : Constant  Value=0
  Constant2 : Constant  Value=CAL_FilterResetThd
  Constant3 : Constant  Value=CONST_EnableDelay
  Divide1 : Product  Inputs=*/  OutDataTypeStr=Inherit: Inherit via back propagation
  MeasurementNoise1 : Constant  Value=CAL_MeasNoiseVelKF
  ProcessNoise1 : Constant  Value=CAL_procNoiseVelKF
  Product4 : Product  OutDataTypeStr=Inherit: Inherit via back propagation
  Product5 : Product  OutDataTypeStr=single
  Product6 : Product  OutDataTypeStr=Inherit: Inherit via back propagation
  Relational Operator : RelationalOperator  Operator=>  OutDataTypeStr=boolean  RndMeth=Nearest
  Subtract : Sum  Inputs=+-
  Subtract2 : Sum  Inputs=-+
  Subtract3 : Sum  Inputs=-+  OutDataTypeStr=Inherit: Inherit via back propagation
  Unit Delay : UnitDelay  InitialCondition=CAL_NORTH  SampleTime=-1
      settings: AttributesFormatString=%<InitialCondition>
  Unit Delay Enabled Resettable1 : simulink_need_slupdate/Unit Delay Enabled Resettable  vinit=1  tsamp=-1
  constant1 : Constant  OutDataTypeStr=single
  " vel_Filtered" : Outport
  wires:
  Constant/1 -> [delayReset]
  Abs/1 -> Relational Operator/1
  [delayReset] -> Unit Delay Enabled Resettable1/3
  Constant3/1 -> Unit Delay Enabled Resettable1/2
  Constant2/1 -> Relational Operator/2
  Subtract/1 -> Abs/1
  Unit Delay/1 -> Subtract/2
  Add4/1 -> " vel_Filtered"/1  "XT"
  Product5/1 -> Add4/2
  Product6/1 -> Unit Delay Enabled Resettable1/1  "PT"
  Subtract3/1 -> Product6/1
  constant1/1 -> Subtract3/2
  Subtract2/1 -> Product5/1
  velEst/1 -> Add4/1, Subtract2/1  "XT-1"
  Divide1/1 -> Product5/2, Subtract3/1  "KT"
  Add3/1 -> Divide1/1
  MeasurementNoise1/1 -> Add3/1
  Product4/1 -> Add3/2, Divide1/2, Product6/2
  Unit Delay Enabled Resettable1/1 -> Product4/2  "PT-1"
  ProcessNoise1/1 -> Product4/1
  velMeas/1 -> Unit Delay/1, Subtract2/2, Subtract/1  "ZT"

== system DSCA/DSCA/VelocityCalculator/LeftVelocityCalculator/LeftMotor/MotorModelEstimator ==
  pos : Inport
  neg : Inport  Port=2
  Add2 : Sum  Inputs=+-  OutDataTypeStr=int16
  Constant : Constant  Value=CAL_WheelDiameter_cm
  Gain : Gain  Gain=12/255  OutDataTypeStr=single
  Gain1 : Gain  Gain=10/2
  Gain3 : Gain  Gain=1/(gearRatio)
  Product : Product
  motorModelTfDis : MotorModelDiscreteTf/motorModelTfDis
  motorSpd : Outport
  wires:
  Gain/1 -> motorModelTfDis/1
  Constant/1 -> Gain1/1
  Gain3/1 -> Product/1  "WmotorGear"
  motorModelTfDis/1 -> Gain3/1  "Wmotor"
  Gain1/1 -> Product/2
  Product/1 -> motorSpd/1
  pos/1 -> Add2/1
  neg/1 -> Add2/2
  Add2/1 -> Gain/1

== system DSCA/DSCA/VelocityCalculator/LeftVelocityCalculator/LeftMotor/VelocityFilter1 ==
  distanceInstant : Inport
  Add4 : Sum  Inputs=+-
  Add5 : Sum
  Data Type Conversion : DataTypeConversion  OutDataTypeStr=single
  Delay : Delay  DelayLength=1
  Delay1 : Delay  DelayLength=1  InitialCondition=single(0)
  Gain3 : Gain  Gain=single(1/1)
  DistTravelled_mm : Outport
  wires:
  Add4/1 -> Add5/1
  Add5/1 -> Delay1/1, Gain3/1
  Delay1/1 -> Add5/2
  Delay/1 -> Add4/2
  Gain3/1 -> Data Type Conversion/1
  distanceInstant/1 -> Add4/1, Delay/1
  Data Type Conversion/1 -> DistTravelled_mm/1

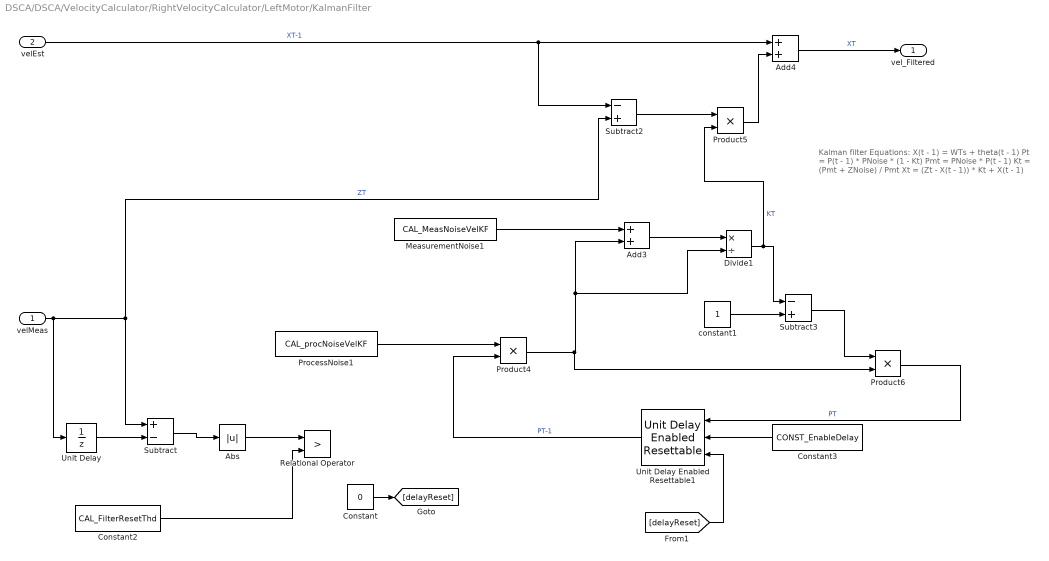
== system DSCA/DSCA/VelocityCalculator/RightVelocityCalculator/LeftMotor/KalmanFilter ==
  note: Kalman filter Equations:
      | X(t - 1) = WTs + theta(t - 1)
      | Pt = P(t - 1) * PNoise * (1 - Kt)
      | Pmt = PNoise * P(t - 1)
      | Kt = (Pmt + ZNoise) / Pmt
      | Xt = (Zt - X(t - 1)) * Kt + X(t - 1)
  velMeas : Inport
  velEst : Inport  Port=2
  Abs : Abs
  Add3 : Sum
  Add4 : Sum  OutDataTypeStr=single
  Constant : Constant  Value=0
  Constant2 : Constant  Value=CAL_FilterResetThd
  Constant3 : Constant  Value=CONST_EnableDelay
  Divide1 : Product  Inputs=*/  OutDataTypeStr=Inherit: Inherit via back propagation
  MeasurementNoise1 : Constant  Value=CAL_MeasNoiseVelKF
  ProcessNoise1 : Constant  Value=CAL_procNoiseVelKF
  Product4 : Product  OutDataTypeStr=Inherit: Inherit via back propagation
  Product5 : Product  OutDataTypeStr=single
  Product6 : Product  OutDataTypeStr=Inherit: Inherit via back propagation
  Relational Operator : RelationalOperator  Operator=>  OutDataTypeStr=boolean  RndMeth=Nearest
  Subtract : Sum  Inputs=+-
  Subtract2 : Sum  Inputs=-+
  Subtract3 : Sum  Inputs=-+  OutDataTypeStr=Inherit: Inherit via back propagation
  Unit Delay : UnitDelay  InitialCondition=CAL_NORTH  SampleTime=-1
      settings: AttributesFormatString=%<InitialCondition>
  Unit Delay Enabled Resettable1 : simulink_need_slupdate/Unit Delay Enabled Resettable  vinit=1  tsamp=-1
  constant1 : Constant  OutDataTypeStr=single
  " vel_Filtered" : Outport
  wires:
  Constant/1 -> [delayReset]
  Abs/1 -> Relational Operator/1
  [delayReset] -> Unit Delay Enabled Resettable1/3
  Constant3/1 -> Unit Delay Enabled Resettable1/2
  Constant2/1 -> Relational Operator/2
  Subtract/1 -> Abs/1
  Unit Delay/1 -> Subtract/2
  Add4/1 -> " vel_Filtered"/1  "XT"
  Product5/1 -> Add4/2
  Product6/1 -> Unit Delay Enabled Resettable1/1  "PT"
  Subtract3/1 -> Product6/1
  constant1/1 -> Subtract3/2
  Subtract2/1 -> Product5/1
  velEst/1 -> Add4/1, Subtract2/1  "XT-1"
  Divide1/1 -> Product5/2, Subtract3/1  "KT"
  Add3/1 -> Divide1/1
  MeasurementNoise1/1 -> Add3/1
  Product4/1 -> Add3/2, Divide1/2, Product6/2
  Unit Delay Enabled Resettable1/1 -> Product4/2  "PT-1"
  ProcessNoise1/1 -> Product4/1
  velMeas/1 -> Unit Delay/1, Subtract2/2, Subtract/1  "ZT"

== system DSCA/DSCA/VelocityCalculator/RightVelocityCalculator/LeftMotor/MotorModelEstimator ==
  pos : Inport
  neg : Inport  Port=2
  Add2 : Sum  Inputs=+-  OutDataTypeStr=int16
  Constant : Constant  Value=CAL_WheelDiameter_cm
  Gain : Gain  Gain=12/255  OutDataTypeStr=single
  Gain1 : Gain  Gain=10/2
  Gain3 : Gain  Gain=1/(gearRatio)
  Product : Product
  motorModelTfDis : MotorModelDiscreteTf/motorModelTfDis
  motorSpd : Outport
  wires:
  Gain/1 -> motorModelTfDis/1
  Constant/1 -> Gain1/1
  Gain3/1 -> Product/1  "WmotorGear"
  motorModelTfDis/1 -> Gain3/1  "Wmotor"
  Gain1/1 -> Product/2
  Product/1 -> motorSpd/1
  pos/1 -> Add2/1
  neg/1 -> Add2/2
  Add2/1 -> Gain/1

== system DSCA/DSCA/VelocityCalculator/RightVelocityCalculator/LeftMotor/VelocityFilter1 ==
  distanceInstant : Inport
  Add4 : Sum  Inputs=+-
  Add5 : Sum
  Data Type Conversion : DataTypeConversion  OutDataTypeStr=single
  Delay : Delay  DelayLength=1
  Delay1 : Delay  DelayLength=1  InitialCondition=single(0)
  Gain3 : Gain  Gain=single(1/1)
  DistTravelled_mm : Outport
  wires:
  Data Type Conversion/1 -> DistTravelled_mm/1
  distanceInstant/1 -> Delay/1, Add4/1
  Gain3/1 -> Data Type Conversion/1
  Delay/1 -> Add4/2
  Delay1/1 -> Add5/2
  Add5/1 -> Gain3/1, Delay1/1
  Add4/1 -> Add5/1

== stateflow chart DSCA/VelocityCalculator/LeftVelocityCalculator/LeftMotor/Chart ==
  state counting
    en:
    cycleCnt = 1;
    du:
    cycleCnt++;
  state stop
    en:
    spd = 0;
  counting -> counting [order 1] : [hasChangedTo(encoderTick, true)]
      | /spd = (CAL_mm_PER_tick / (cycleCnt * CAL_EncoderSampleTime));
  (default) -> counting
  stop -> counting : [hasChanged(encoderTick)]
  counting -> stop [order 2] : [cycleCnt > (100)]
  data: CAL_EncoderSampleTime constant single =CAL_EncoderSampleTime; spd output single; cycleCnt local uint8; encoderTick input; CAL_mm_PER_tick constant single =CAL_mm_PER_tick

== stateflow chart DSCA/VelocityCalculator/RightVelocityCalculator/LeftMotor/Chart ==
  state counting
    en:
    cycleCnt = 1;
    du:
    cycleCnt++;
  state stop
    en:
    spd = 0;
  counting -> counting [order 1] : [hasChangedTo(encoderTick, true)]
      | /spd = (CAL_mm_PER_tick / (cycleCnt * CAL_EncoderSampleTime));
  (default) -> counting
  stop -> counting : [hasChanged(encoderTick)]
  counting -> stop [order 2] : [cycleCnt > (100)]
  data: CAL_EncoderSampleTime constant single =CAL_EncoderSampleTime; spd output single; cycleCnt local uint8; encoderTick input; CAL_mm_PER_tick constant single =CAL_mm_PER_tick

== stateflow chart DSCA/Encoder_endofLineTest/endofLineTest/Chart ==
  state InitializeTest
    en:
    EOL_leftMoveReq = ENU_STOP;
    EOL_rightMoveReq = ENU_STOP;
    counterReset = true;
  state SlowPwm
  state MediumPwm
    on after(CONST_EnDelay, tick):
    counterReset = false;
    EOL_pwm = CONST_EOL_MedPwm;
    EOL_leftMoveReq = ENU_FORWARD;
    EOL_rightMoveReq = ENU_FORWARD;
  state SuperFastPwm
    on after(CONST_EnDelay, tick):
    counterReset = false;
    EOL_pwm = CONST_EOL_SFastPwm;
    EOL_leftMoveReq = ENU_FORWARD;
    EOL_rightMoveReq = ENU_FORWARD;
  state FastPwm
    on after(CONST_EnDelay, tick):
    counterReset = false;
    EOL_pwm = CONST_EOL_FastPwm;
    EOL_leftMoveReq = ENU_FORWARD;
    EOL_rightMoveReq = ENU_FORWARD;
  (default) -> InitializeTest
  SlowPwm -> MediumPwm : [leftEncoderCounter_uint16 >= CONST_EOL_ME_Ticks]
      | /EOL_leftMoveReq = ENU_STOP;
      | EOL_rightMoveReq = ENU_STOP;
      | counterReset = true;
  InitializeTest -> SlowPwm : [after(CONST_EnDelay, tick)]
      | /counterReset = false;
      | EOL_pwm = CONST_EOL_SlowPwm;
      | EOL_leftMoveReq = ENU_FORWARD;
      | EOL_rightMoveReq = ENU_FORWARD;
  SuperFastPwm -> InitializeTest : [leftEncoderCounter_uint16 >= CONST_EOL_ME_Ticks]
  MediumPwm -> FastPwm : [leftEncoderCounter_uint16 >= CONST_EOL_ME_Ticks]
      | /EOL_leftMoveReq = ENU_STOP;
      | EOL_rightMoveReq = ENU_STOP;
      | counterReset = true;
  FastPwm -> SuperFastPwm : [leftEncoderCounter_uint16 >= CONST_EOL_ME_Ticks]
      | /EOL_leftMoveReq = ENU_STOP;
      | EOL_rightMoveReq = ENU_STOP;
      | counterReset = true;
  data: CONST_EnDelay constant uint16 =CONST_EnDelay; EOL_pwm output single; EOL_leftMoveReq output uint8; EOL_rightMoveReq output uint8; leftEncoderCounter_uint16 input; rightEncoderCounter_uint16 input; CONST_EOL_FastPwm constant uint8 =CONST_EOL_FastPwm; CONST_EOL_ME_Ticks constant uint16 =CONST_EOL_ME_Ticks; CONST_EOL_MedPwm constant uint8 =CONST_EOL_MedPwm; CONST_EOL_SFastPwm constant uint8 =CONST_EOL_SFastPwm; CONST_EOL_SlowPwm constant uint8 =CONST_EOL_SlowPwm; ENU_FORWARD constant double =ENU_FORWARD; ENU_STOP constant double =ENU_STOP; counterReset output double
